simulink model "manufacturing"  (R2016a)
settings: Solver=FixedStepAuto  StartTime=0.0  StopTime=40  FixedStep=1  RelTol=1e-3
values from neighbouring files (symbols this model uses):
  averaging = 8    [parameters.m]    (also in preprocessing.m)
  first_initialcapacity = 0.6    [parameters.m]
  first_processtime = 1.5    [parameters.m]
  initialorder = 10000    [parameters.m]    (also in preprocessing.m)
  inventoryadjustment = 8    [parameters.m]    (also in preprocessing.m)
  second_initialcapacity = 0.6    [parameters.m]
  second_processtime = 1.5    [parameters.m]
  targetdeliverydelay = 2    [parameters.m]    (also in preprocessing.m)
  third_initialcapacity = 0.6    [parameters.m]
  third_processtime = 1.5    [parameters.m]
  totalcycletime = (first_processtime+second_processtime+third_processtime)*3/2    (= 6.75)    [parameters.m]    (also in preprocessing.m)
  wipadjustment = 2    [parameters.m]    (also in preprocessing.m)
undefined symbols (not defined in the file or in its folder): magnitude
settings Model: Creator=yshun  LastModifiedBy=yshun
settings DataIOCC: SaveFormat=Array

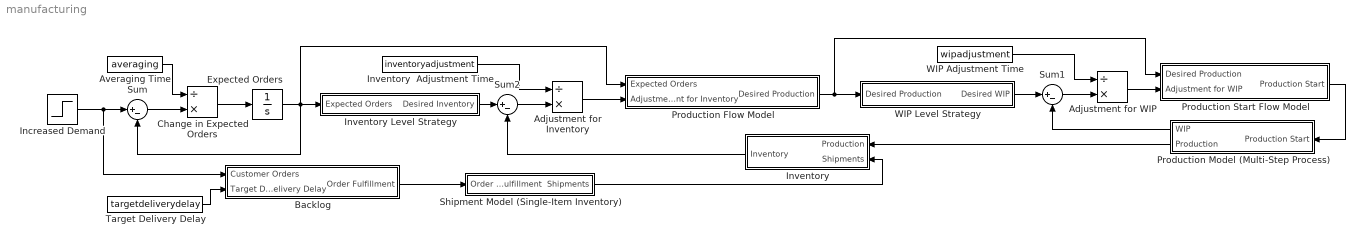
== system manufacturing ==
  Adjustment for Inventory : Product  Inputs=/*
  Adjustment for WIP : Product  Inputs=/*
  Averaging Time : Constant  Value=averaging
  Backlog : Subsystem
  Change in Expected Orders : Product  Inputs=/*
  Expected Orders : Integrator  InitialCondition=10000
  Increased Demand : Step  Time=5  Before=initialorder  After=12000  SampleTime=0
  Inventory : Subsystem
  Inventory  Adjustment Time : Constant  Value=inventoryadjustment
  Inventory Level Strategy : Subsystem
  Production Flow Model : Subsystem
  Production Model (Multi-Step Process) : Subsystem
  Production Start Flow Model : Subsystem
  Shipment Model (Single-Item Inventory) : Subsystem
  Sum : Sum  Inputs=|+-
  Sum1 : Sum  Inputs=|+-
  Sum2 : Sum  Inputs=|+-
  Target Delivery Delay : Constant  Value=targetdeliverydelay
  WIP Adjustment Time : Constant  Value=wipadjustment
  WIP Level Strategy : Subsystem
  wires:
  Sum/1 -> Change in Expected Orders/2
  Expected Orders/1 -> Sum/2, Production Flow Model/1(Expected Orders), Inventory Level Strategy/1(Expected Orders)
  Inventory Level Strategy/1(Desired Inventory) -> Sum2/1
  Change in Expected Orders/1 -> Expected Orders/1
  Sum2/1 -> Adjustment for Inventory/2
  Adjustment for Inventory/1 -> Production Flow Model/2(Adjustment for Inventory)
  Sum1/1 -> Adjustment for WIP/2
  WIP Level Strategy/1(Desired WIP) -> Sum1/1
  Production Flow Model/1(Desired Production) -> WIP Level Strategy/1(Desired Production), Production Start Flow Model/1("Desired Production ")
  Adjustment for WIP/1 -> Production Start Flow Model/2(Adjustment for WIP)
  Production Start Flow Model/1(Production Start) -> Production Model (Multi-Step Process)/1(Production Start)
  Production Model (Multi-Step Process)/2(Production) -> Inventory/1(Production)
  Inventory/1(Inventory) -> Sum2/2
  Production Model (Multi-Step Process)/1(WIP) -> Sum1/2
  Increased Demand/1 -> Backlog/1(Customer Orders), Sum/1
  Backlog/1(Order Fulfillment) -> Shipment Model (Single-Item Inventory)/1(Order Fulfillment)
  Shipment Model (Single-Item Inventory)/1(Shipments) -> Inventory/2(Shipments)
  Averaging Time/1 -> Change in Expected Orders/1
  Inventory  Adjustment Time/1 -> Adjustment for Inventory/1
  WIP Adjustment Time/1 -> Adjustment for WIP/1
  Target Delivery Delay/1 -> Backlog/2(Target Delivery Delay)

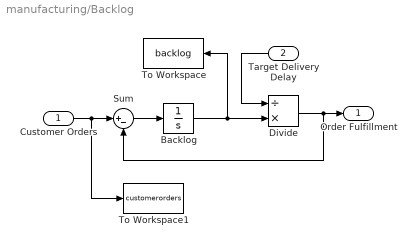
== system manufacturing/Backlog ==
  Customer Orders : Inport
  Target Delivery Delay : Inport  Port=2
  Backlog : Integrator  InitialCondition=20000
  Divide : Product  Inputs=/*
  Sum : Sum  Inputs=|+-
  To Workspace : ToWorkspace  VariableName=backlog  SaveFormat=Timeseries  SampleTime=-1
  To Workspace1 : ToWorkspace  VariableName=customerorders  SaveFormat=Timeseries  SampleTime=-1
  Order Fulfillment : Outport
  wires:
  Divide/1 -> Sum/2, Order Fulfillment/1
  Customer Orders/1 -> To Workspace1/1, Sum/1
  Sum/1 -> Backlog/1
  Backlog/1 -> To Workspace/1, Divide/2
  Target Delivery Delay/1 -> Divide/1

== system manufacturing/Inventory ==
  Production : Inport
  Shipments : Inport  Port=2
  Add : Sum  Inputs=+-
  Integrator : Integrator  InitialCondition=40000
  To Workspace : ToWorkspace  VariableName=inventory  SaveFormat=Timeseries  SampleTime=-1
  Inventory : Outport
  wires:
  Production/1 -> Add/1
  Shipments/1 -> Add/2
  Add/1 -> Integrator/1
  Integrator/1 -> To Workspace/1, Inventory/1

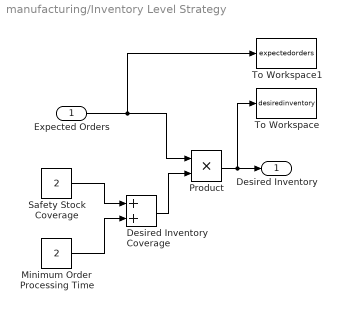
== system manufacturing/Inventory Level Strategy ==
  Expected Orders : Inport
  Desired Inventory Coverage : Sum
  Minimum Order Processing Time : Constant  Value=2
  Product : Product
  Safety Stock Coverage : Constant  Value=2
  To Workspace : ToWorkspace  VariableName=desiredinventory  SaveFormat=Timeseries  SampleTime=-1
  To Workspace1 : ToWorkspace  VariableName=expectedorders  SaveFormat=Timeseries  SampleTime=-1
  Desired Inventory : Outport
  wires:
  Safety Stock Coverage/1 -> Desired Inventory Coverage/1
  Minimum Order Processing Time/1 -> Desired Inventory Coverage/2
  Expected Orders/1 -> Product/1, To Workspace1/1
  Desired Inventory Coverage/1 -> Product/2
  Product/1 -> To Workspace/1, Desired Inventory/1

== system manufacturing/Production Flow Model ==
  Expected Orders : Inport
  Adjustment for Inventory : Inport  Port=2
  Add : Sum
  Constant : Constant  Value=0
  MinMax : MinMax  Function=max  Inputs=2
  To Workspace : ToWorkspace  VariableName=desiredproduction  SaveFormat=Timeseries  SampleTime=-1
  Desired Production : Outport
  wires:
  Expected Orders/1 -> Add/1
  Adjustment for Inventory/1 -> Add/2
  Add/1 -> MinMax/1
  Constant/1 -> MinMax/2
  MinMax/1 -> To Workspace/1, Desired Production/1

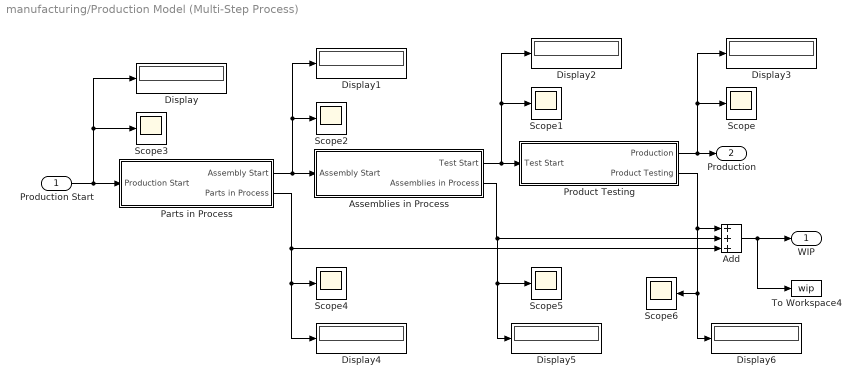
== system manufacturing/Production Model (Multi-Step Process) ==
  Production Start : Inport
  Add : Sum  Inputs=+++
  Assemblies in Process : Subsystem
  Display{,1..6} (7 alike) : Display
  Parts in Process : Subsystem
  Product Testing : Subsystem
  Scope{,1..6} (7 alike) : Scope
  To Workspace4 : ToWorkspace  VariableName=wip  SaveFormat=Timeseries  SampleTime=-1
  WIP : Outport
  Production : Outport  Port=2
  wires:
  Production Start/1 -> Display/1, Scope3/1, Parts in Process/1(Production Start)
  Parts in Process/1(Assembly Start) -> Display1/1, Scope2/1, Assemblies in Process/1(Assembly Start)
  Add/1 -> To Workspace4/1, WIP/1
  Parts in Process/2(Parts in Process) -> Display4/1, Scope4/1, Add/3
  Assemblies in Process/2(Assemblies in Process) -> Display5/1, Scope5/1, Add/2
  Assemblies in Process/1(Test Start) -> Display2/1, Scope1/1, Product Testing/1(Test Start)
  Product Testing/2(Product Testing) -> Display6/1, Scope6/1, Add/1
  Product Testing/1(Production) -> Display3/1, Scope/1, Production/1

== system manufacturing/Production Start Flow Model ==
  "Desired Production " : Inport
  Adjustment for WIP : Inport  Port=2
  Add : Sum
  Constant : Constant  Value=0
  MinMax : MinMax  Function=max  Inputs=2
  To Workspace : ToWorkspace  VariableName=productionstart  SaveFormat=Timeseries  SampleTime=-1
  Production Start : Outport
  wires:
  "Desired Production "/1 -> Add/1
  Adjustment for WIP/1 -> Add/2
  Add/1 -> MinMax/1
  Constant/1 -> MinMax/2
  MinMax/1 -> To Workspace/1, Production Start/1

== system manufacturing/Shipment Model (Single-Item Inventory) ==
  Order Fulfillment : Inport
  To Workspace : ToWorkspace  VariableName=shipments  SaveFormat=Timeseries  SampleTime=-1
  Shipments : Outport
  wires:
  Order Fulfillment/1 -> Shipments/1, To Workspace/1

== system manufacturing/WIP Level Strategy ==
  Desired Production : Inport
  Constant : Constant  Value=totalcycletime
  Product : Product
  To Workspace : ToWorkspace  VariableName=desiredwip  SaveFormat=Timeseries  SampleTime=-1
  Desired WIP : Outport
  wires:
  Desired Production/1 -> Product/2
  Product/1 -> To Workspace/1, Desired WIP/1
  Constant/1 -> Product/1

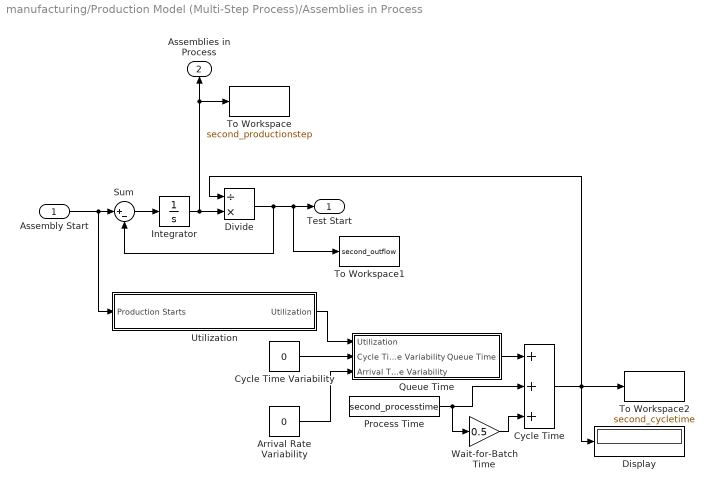
== system manufacturing/Production Model (Multi-Step Process)/Assemblies in Process ==
  Assembly Start : Inport
  Arrival Rate Variability : Constant  Value=0
  Cycle Time : Sum  Inputs=+++
  Cycle Time Variability : Constant  Value=0
  Display : Display
  Divide : Product  Inputs=/*
  Integrator : Integrator  InitialCondition=initialorder*totalcycletime/3
  Process Time : Constant  Value=second_processtime
  Queue Time : Subsystem
  Sum : Sum  Inputs=|+-
  To Workspace : ToWorkspace  VariableName=second_productionstep  SaveFormat=Timeseries  SampleTime=-1
  To Workspace1 : ToWorkspace  VariableName=second_outflow  SaveFormat=Timeseries  SampleTime=-1
  To Workspace2 : ToWorkspace  VariableName=second_cycletime  SaveFormat=Timeseries  SampleTime=-1
  Utilization : Subsystem
  Wait-for-Batch Time : Gain  Gain=0.5
  Test Start : Outport
  Assemblies in Process : Outport  Port=2
  wires:
  Assembly Start/1 -> Utilization/1(Production Starts), Sum/1
  Sum/1 -> Integrator/1
  Integrator/1 -> To Workspace/1, Assemblies in Process/1, Divide/2
  Divide/1 -> To Workspace1/1, Test Start/1, Sum/2
  Utilization/1(Utilization) -> Queue Time/1(Utilization)
  Cycle Time Variability/1 -> Queue Time/2(Cycle Time Variability)
  Arrival Rate Variability/1 -> Queue Time/3(Arrival Time Variability)
  Cycle Time/1 -> Divide/1, To Workspace2/1, Display/1
  Wait-for-Batch Time/1 -> Cycle Time/3
  Queue Time/1(Queue Time) -> Cycle Time/1
  Process Time/1 -> Cycle Time/2, Wait-for-Batch Time/1

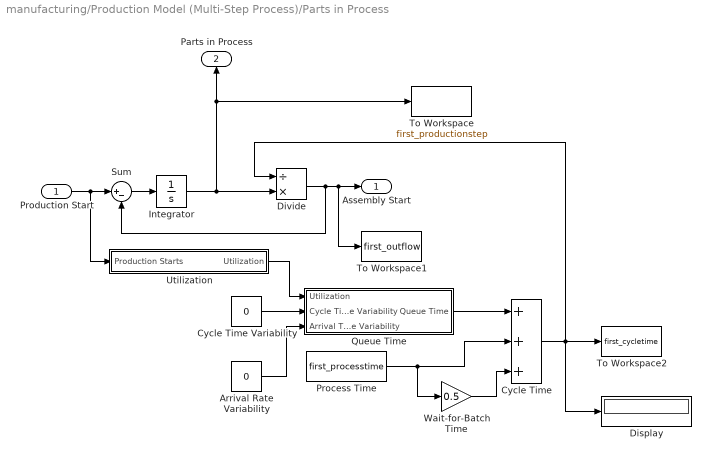
== system manufacturing/Production Model (Multi-Step Process)/Parts in Process ==
  Production Start : Inport
  Arrival Rate Variability : Constant  Value=0
  Cycle Time : Sum  Inputs=+++
  Cycle Time Variability : Constant  Value=0
  Display : Display
  Divide : Product  Inputs=/*
  Integrator : Integrator  InitialCondition=initialorder*totalcycletime/3
  Process Time : Constant  Value=first_processtime
  Queue Time : Subsystem
  Sum : Sum  Inputs=|+-
  To Workspace : ToWorkspace  VariableName=first_productionstep  SaveFormat=Timeseries  SampleTime=-1
  To Workspace1 : ToWorkspace  VariableName=first_outflow  SaveFormat=Timeseries  SampleTime=-1
  To Workspace2 : ToWorkspace  VariableName=first_cycletime  SaveFormat=Timeseries  SampleTime=-1
  Utilization : Subsystem
  Wait-for-Batch Time : Gain  Gain=0.5
  Assembly Start : Outport
  Parts in Process : Outport  Port=2
  wires:
  Production Start/1 -> Utilization/1(Production Starts), Sum/1
  Sum/1 -> Integrator/1
  Integrator/1 -> Divide/2, Parts in Process/1, To Workspace/1
  Divide/1 -> Sum/2, To Workspace1/1, Assembly Start/1
  Utilization/1(Utilization) -> Queue Time/1(Utilization)
  Cycle Time Variability/1 -> Queue Time/2(Cycle Time Variability)
  Arrival Rate Variability/1 -> Queue Time/3(Arrival Time Variability)
  Queue Time/1(Queue Time) -> Cycle Time/1
  Process Time/1 -> Cycle Time/2, Wait-for-Batch Time/1
  Cycle Time/1 -> Display/1, Divide/1, To Workspace2/1
  Wait-for-Batch Time/1 -> Cycle Time/3

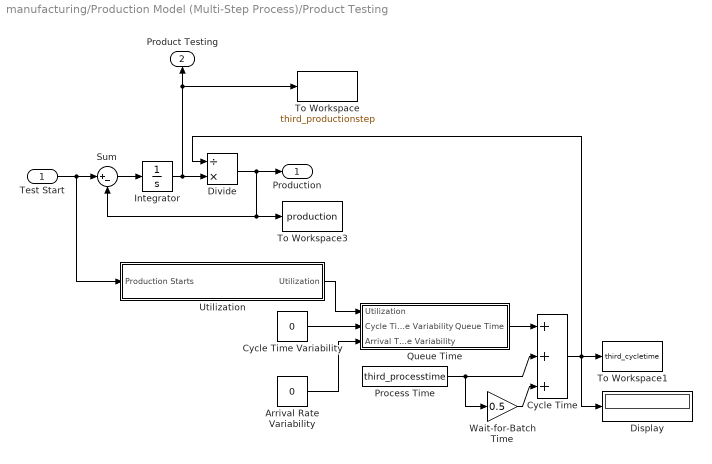
== system manufacturing/Production Model (Multi-Step Process)/Product Testing ==
  Test Start : Inport
  Arrival Rate Variability : Constant  Value=0
  Cycle Time : Sum  Inputs=+++
  Cycle Time Variability : Constant  Value=0
  Display : Display
  Divide : Product  Inputs=/*
  Integrator : Integrator  InitialCondition=initialorder*totalcycletime/3
  Process Time : Constant  Value=third_processtime
  Queue Time : Subsystem
  Sum : Sum  Inputs=|+-
  To Workspace : ToWorkspace  VariableName=third_productionstep  SaveFormat=Timeseries  SampleTime=-1
  To Workspace1 : ToWorkspace  VariableName=third_cycletime  SaveFormat=Timeseries  SampleTime=-1
  To Workspace3 : ToWorkspace  VariableName=production  SaveFormat=Timeseries  SampleTime=-1
  Utilization : Subsystem
  Wait-for-Batch Time : Gain  Gain=0.5
  Production : Outport
  Product Testing : Outport  Port=2
  wires:
  Test Start/1 -> Utilization/1(Production Starts), Sum/1
  Sum/1 -> Integrator/1
  Integrator/1 -> Product Testing/1, To Workspace/1, Divide/2
  Divide/1 -> Production/1, Sum/2, To Workspace3/1
  Utilization/1(Utilization) -> Queue Time/1(Utilization)
  Cycle Time Variability/1 -> Queue Time/2(Cycle Time Variability)
  Arrival Rate Variability/1 -> Queue Time/3(Arrival Time Variability)
  Queue Time/1(Queue Time) -> Cycle Time/1
  Wait-for-Batch Time/1 -> Cycle Time/3
  Cycle Time/1 -> Display/1, Divide/1, To Workspace1/1
  Process Time/1 -> Wait-for-Batch Time/1, Cycle Time/2

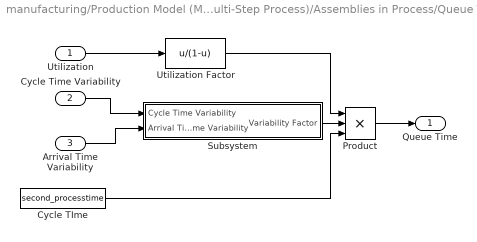
== system manufacturing/Production Model (Multi-Step Process)/Assemblies in Process/Queue Time ==
  Utilization : Inport
  Cycle Time Variability : Inport  Port=2
  Arrival Time Variability : Inport  Port=3
  Cycle TIme : Constant  Value=second_processtime
  Product : Product  Inputs=3
  Subsystem : Subsystem
  Utilization Factor : Fcn  Expr=u/(1-u)
  Queue Time : Outport
  wires:
  Utilization/1 -> Utilization Factor/1
  Cycle Time Variability/1 -> Subsystem/1(Cycle Time Variability)
  Arrival Time Variability/1 -> Subsystem/2(Arrival Time Variability)
  Utilization Factor/1 -> Product/1
  Subsystem/1(Variability Factor) -> Product/2
  Cycle TIme/1 -> Product/3
  Product/1 -> Queue Time/1

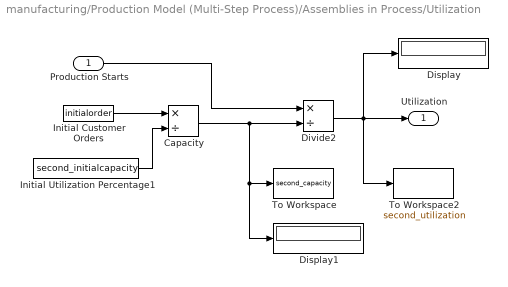
== system manufacturing/Production Model (Multi-Step Process)/Assemblies in Process/Utilization ==
  Production Starts : Inport
  Capacity : Product  Inputs=*/
  Display : Display
  Display1 : Display
  Divide2 : Product  Inputs=*/
  Initial Customer Orders : Constant  Value=initialorder
  Initial Utilization Percentage1 : Constant  Value=second_initialcapacity
  To Workspace : ToWorkspace  VariableName=second_capacity  SaveFormat=Timeseries  SampleTime=-1
  To Workspace2 : ToWorkspace  VariableName=second_utilization  SaveFormat=Timeseries  SampleTime=-1
  Utilization : Outport
  wires:
  Divide2/1 -> To Workspace2/1, Display/1, Utilization/1
  Initial Customer Orders/1 -> Capacity/1
  Capacity/1 -> Display1/1, To Workspace/1, Divide2/2
  Production Starts/1 -> Divide2/1
  Initial Utilization Percentage1/1 -> Capacity/2

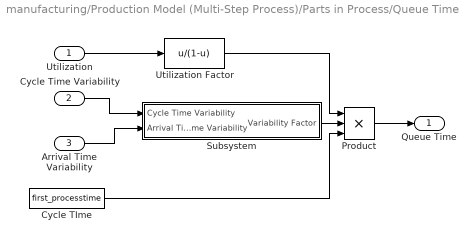
== system manufacturing/Production Model (Multi-Step Process)/Parts in Process/Queue Time ==
  Utilization : Inport
  Cycle Time Variability : Inport  Port=2
  Arrival Time Variability : Inport  Port=3
  Cycle TIme : Constant  Value=first_processtime
  Product : Product  Inputs=3
  Subsystem : Subsystem
  Utilization Factor : Fcn  Expr=u/(1-u)
  Queue Time : Outport
  wires:
  Utilization/1 -> Utilization Factor/1
  Cycle Time Variability/1 -> Subsystem/1(Cycle Time Variability)
  Arrival Time Variability/1 -> Subsystem/2(Arrival Time Variability)
  Utilization Factor/1 -> Product/1
  Subsystem/1(Variability Factor) -> Product/2
  Cycle TIme/1 -> Product/3
  Product/1 -> Queue Time/1

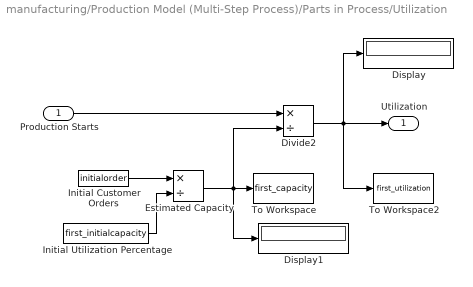
== system manufacturing/Production Model (Multi-Step Process)/Parts in Process/Utilization ==
  Production Starts : Inport
  Display : Display
  Display1 : Display
  Divide2 : Product  Inputs=*/
  Estimated Capacity : Product  Inputs=*/
  Initial Customer Orders : Constant  Value=initialorder
  Initial Utilization Percentage : Constant  Value=first_initialcapacity
  To Workspace : ToWorkspace  VariableName=first_capacity  SaveFormat=Timeseries  SampleTime=-1
  To Workspace2 : ToWorkspace  VariableName=first_utilization  SaveFormat=Timeseries  SampleTime=-1
  Utilization : Outport
  wires:
  Divide2/1 -> To Workspace2/1, Display/1, Utilization/1
  Initial Customer Orders/1 -> Estimated Capacity/1
  Production Starts/1 -> Divide2/1
  Initial Utilization Percentage/1 -> Estimated Capacity/2
  Estimated Capacity/1 -> Display1/1, Divide2/2, To Workspace/1

== system manufacturing/Production Model (Multi-Step Process)/Product Testing/Queue Time ==
  Utilization : Inport
  Cycle Time Variability : Inport  Port=2
  Arrival Time Variability : Inport  Port=3
  Cycle TIme : Constant  Value=third_processtime
  Product : Product  Inputs=3
  Subsystem : Subsystem
  Utilization Factor : Fcn  Expr=u/(1-u)
  Queue Time : Outport
  wires:
  Utilization/1 -> Utilization Factor/1
  Cycle Time Variability/1 -> Subsystem/1(Cycle Time Variability)
  Arrival Time Variability/1 -> Subsystem/2(Arrival Time Variability)
  Utilization Factor/1 -> Product/1
  Subsystem/1(Variability Factor) -> Product/2
  Cycle TIme/1 -> Product/3
  Product/1 -> Queue Time/1

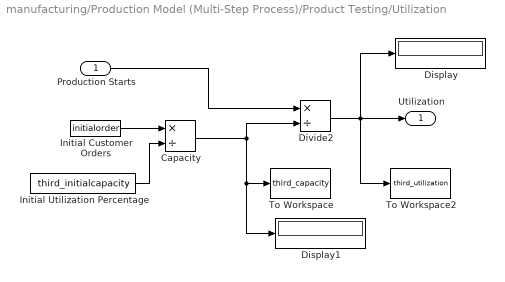
== system manufacturing/Production Model (Multi-Step Process)/Product Testing/Utilization ==
  Production Starts : Inport
  Capacity : Product  Inputs=*/
  Display : Display
  Display1 : Display
  Divide2 : Product  Inputs=*/
  Initial Customer Orders : Constant  Value=initialorder
  Initial Utilization Percentage : Constant  Value=third_initialcapacity
  To Workspace : ToWorkspace  VariableName=third_capacity  SaveFormat=Timeseries  SampleTime=-1
  To Workspace2 : ToWorkspace  VariableName=third_utilization  SaveFormat=Timeseries  SampleTime=-1
  Utilization : Outport
  wires:
  Divide2/1 -> To Workspace2/1, Display/1, Utilization/1
  Initial Customer Orders/1 -> Capacity/1
  Capacity/1 -> Divide2/2, Display1/1, To Workspace/1
  Production Starts/1 -> Divide2/1
  Initial Utilization Percentage/1 -> Capacity/2

== system manufacturing/Production Model (Multi-Step Process)/Assemblies in Process/Queue Time/Subsystem ==
  Cycle Time Variability : Inport
  Arrival Time Variability : Inport  Port=2
  Add : Sum
  Constant : Constant  Value=2
  Divide : Product  Inputs=*/
  Math Function : Math  Operator=magnitude^2  SaturateOnIntegerOverflow=on
  Math Function1 : Math  Operator=magnitude^2  SaturateOnIntegerOverflow=on
  Variability Factor : Outport
  wires:
  Cycle Time Variability/1 -> Math Function/1
  Arrival Time Variability/1 -> Math Function1/1
  Math Function/1 -> Add/1
  Math Function1/1 -> Add/2
  Add/1 -> Divide/1
  Constant/1 -> Divide/2
  Divide/1 -> Variability Factor/1

== system manufacturing/Production Model (Multi-Step Process)/Parts in Process/Queue Time/Subsystem ==
  Cycle Time Variability : Inport
  Arrival Time Variability : Inport  Port=2
  Add : Sum
  Constant : Constant  Value=2
  Divide : Product  Inputs=*/
  Math Function : Math  Operator=magnitude^2  SaturateOnIntegerOverflow=on
  Math Function1 : Math  Operator=magnitude^2  SaturateOnIntegerOverflow=on
  Variability Factor : Outport
  wires:
  Cycle Time Variability/1 -> Math Function/1
  Arrival Time Variability/1 -> Math Function1/1
  Math Function/1 -> Add/1
  Math Function1/1 -> Add/2
  Add/1 -> Divide/1
  Constant/1 -> Divide/2
  Divide/1 -> Variability Factor/1

== system manufacturing/Production Model (Multi-Step Process)/Product Testing/Queue Time/Subsystem ==
  Cycle Time Variability : Inport
  Arrival Time Variability : Inport  Port=2
  Add : Sum
  Constant : Constant  Value=2
  Divide : Product  Inputs=*/
  Math Function : Math  Operator=magnitude^2  SaturateOnIntegerOverflow=on
  Math Function1 : Math  Operator=magnitude^2  SaturateOnIntegerOverflow=on
  Variability Factor : Outport
  wires:
  Cycle Time Variability/1 -> Math Function/1
  Arrival Time Variability/1 -> Math Function1/1
  Math Function/1 -> Add/1
  Math Function1/1 -> Add/2
  Add/1 -> Divide/1
  Constant/1 -> Divide/2
  Divide/1 -> Variability Factor/1
